simulink model "zad_no_8"  (R2017b)
settings: Solver=VariableStepAuto  StartTime=0.0  StopTime=10.0  RelTol=1e-3
undefined symbols (not defined in the file): Tp, u_c
settings Model: Creator=micha  LastModifiedBy=micha

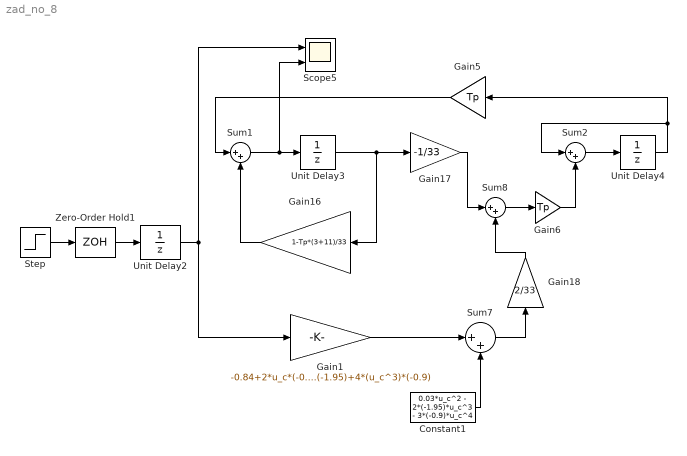
== system zad_no_8 ==
  Constant1 : Constant  Value=0.03*u_c^2 - 2*(-1.95)*u_c^3 - 3*(-0.9)*u_c^4
  Gain1 : Gain  Gain=-0.84+2*u_c*(-0.03)+3*(u_c^2)*(-1.95)+4*(u_c^3)*(-0.9)
  Gain16 : Gain  Gain=1-Tp*(3+11)/33  ParamDataTypeStr=double
  Gain17 : Gain  Gain=-1/33
  Gain18 : Gain  Gain=2/33
  Gain5 : Gain  Gain=Tp  ParamDataTypeStr=double
  Gain6 : Gain  Gain=Tp
  Scope5 : Scope  NumInputPorts=2
  Step : Step  SampleTime=0
  Sum{1..2,7..8} (4 alike) : Sum  Inputs=|++
  Unit Delay2 : UnitDelay  SampleTime=Tp
  Unit Delay3 : UnitDelay  SampleTime=Tp
  Unit Delay4 : UnitDelay  SampleTime=Tp
  Zero-Order Hold1 : ZeroOrderHold  SampleTime=Tp
  wires:
  Gain17/1 -> Sum8/1
  Sum2/1 -> Unit Delay4/1
  Gain18/1 -> Sum8/2
  Sum1/1 -> Scope5/2, Unit Delay3/1
  Unit Delay3/1 -> Gain17/1, Gain16/1
  Unit Delay4/1 -> Gain5/1, Sum2/1
  Gain5/1 -> Sum1/1
  Gain16/1 -> Sum1/2
  Gain1/1 -> Sum7/1
  Constant1/1 -> Sum7/2
  Gain6/1 -> Sum2/2
  Sum8/1 -> Gain6/1
  Sum7/1 -> Gain18/1
  Unit Delay2/1 -> Gain1/1, Scope5/1
  Step/1 -> Zero-Order Hold1/1
  Zero-Order Hold1/1 -> Unit Delay2/1
